simulink model "ObsPertContinuo"  (R2022b)
settings: Solver=ode45  StartTime=0.0  StopTime=700  RelTol=1e-3  EnableMultiTasking=on
settings Model: Creator=adolfobs  LastModifiedBy=adolfo
settings SolverCC: AlgebraicLoopSolver=TrustRegion
settings DataIOCC: LimitDataPoints=on  MaxDataPoints=25000  SaveFormat=Array  SignalLoggingSaveFormat=ModelDataLogs  ReturnWorkspaceOutputs=off
settings OptimizationCC: BlockReduction=off  BooleanDataType=off  InitFltsAndDblsToZero=on  LifeSpan=inf
settings DebuggingCC: SaveWithParameterizedLinksMsg=none  UnderspecifiedInitializationDetection=Classic  MergeDetectMultiDrivingBlocksExec=none  SignalResolutionControl=TryResolveAllWithWarning  MultiTaskDSMMsg=warning  MultiTaskCondExecSysMsg=none  UnconnectedInputMsg=warning  UnconnectedOutputMsg=warning  UnconnectedLineMsg=warning  SFUnexpectedBacktrackingDiag=warning  SFNoUnconditionalDefaultTransitionDiag=warning  SFExecutionAtInitializationDiag=none  SFMachineParentedDataDiag=warning  ArithmeticOperatorsInVariantConditions=warning
settings HardwareCC: ProdBitPerPointer=32  ProdBitPerSizeT=32  ProdBitPerPtrDiffT=32  ProdLargestAtomicFloat=None  ProdIntDivRoundTo=Undefined  ProdEndianess=Unspecified  ProdWordSize=32  ProdHWDeviceType=32-bit Generic  TargetUnknown=on
settings ModelReferenceCC: EnableRefExpFcnMdlSchedulingChecks=on  PropagateSignalLabelsOutOfModel=off
settings SFSimCC: SimUseLocalCustomCode=off  CustomCodeUndefinedFunction=UseInterfaceOnly
settings RTWCC: RTWUseLocalCustomCode=off
settings CodeAppCC: StateflowObjectComments=on
settings GRTTargetCC: TargetFcnLib=ansi_tfl_tmw.mat  TargetLangStandard=C89/C90 (ANSI)  CombineOutputUpdateFcns=off  GRTInterface=on
settings ConfigComp: CovMetricSettings=dw  CovSaveCumulativeToWorkspaceVar=on  CovSaveSingleToWorkspaceVar=on  CovExternalEMLEnable=off

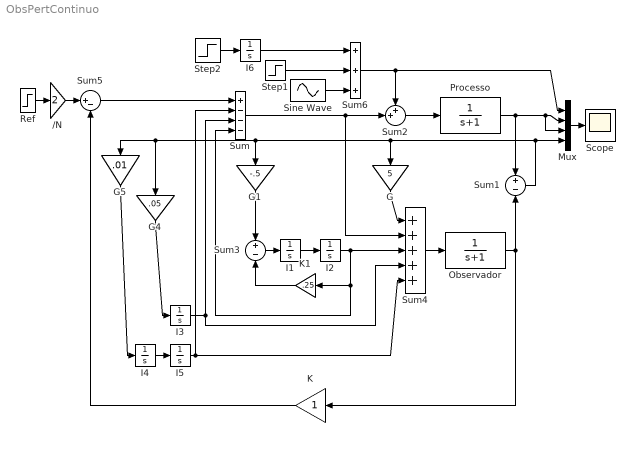
== system ObsPertContinuo ==
  " /N" : Gain  Gain=2  SaturateOnIntegerOverflow=on  OutDataTypeStr=Inherit: Same as input  ParamDataTypeStr=Inherit: Same as input
  G : Gain  Gain=5  SaturateOnIntegerOverflow=on  OutDataTypeStr=Inherit: Same as input  ParamDataTypeStr=Inherit: Same as input
  G1 : Gain  Gain=-.5  SaturateOnIntegerOverflow=on  OutDataTypeStr=Inherit: Same as input  ParamDataTypeStr=Inherit: Same as input
  G4 : Gain  Gain=.05  SaturateOnIntegerOverflow=on  OutDataTypeStr=Inherit: Same as input  ParamDataTypeStr=Inherit: Same as input
  G5 : Gain  Gain=.01  SaturateOnIntegerOverflow=on  OutDataTypeStr=Inherit: Same as input  ParamDataTypeStr=Inherit: Same as input
  I{1..6} (6 alike) : Integrator
  K : Gain  SaturateOnIntegerOverflow=on  OutDataTypeStr=Inherit: Same as input  ParamDataTypeStr=Inherit: Same as input
  K1 : Gain  Gain=.25  SaturateOnIntegerOverflow=on  OutDataTypeStr=Inherit: Same as input  ParamDataTypeStr=Inherit: Same as input
  Mux : Mux
  Observador : TransferFcn  Denominator=[1 1]
  Processo : TransferFcn  Denominator=[1 1]
  Ref : Step  Time=100
  Scope : Scope
  Sine Wave : Sin  Amplitude=.3  Frequency=.5
  Step1 : Step  Time=140  After=.2
  Step2 : Step  Time=400  After=.01
  Sum : Sum  Inputs=+---  InputSameDT=on  SaturateOnIntegerOverflow=on  OutDataTypeStr=Inherit: Same as first input
  Sum1 : Sum  Inputs=+-  InputSameDT=on  SaturateOnIntegerOverflow=on  OutDataTypeStr=Inherit: Same as first input
  Sum2 : Sum  Inputs=++|  InputSameDT=on  SaturateOnIntegerOverflow=on  OutDataTypeStr=Inherit: Same as first input
  Sum3 : Sum  Inputs=+|-  InputSameDT=on  SaturateOnIntegerOverflow=on  OutDataTypeStr=Inherit: Same as first input
  Sum4 : Sum  Inputs=+++++  InputSameDT=on  SaturateOnIntegerOverflow=on  OutDataTypeStr=Inherit: Same as first input
  Sum5 : Sum  Inputs=|+-  InputSameDT=on  SaturateOnIntegerOverflow=on  OutDataTypeStr=Inherit: Same as first input
  Sum6 : Sum  Inputs=+++  InputSameDT=on  SaturateOnIntegerOverflow=on  OutDataTypeStr=Inherit: Same as first input
  wires:
  Sum2/1 -> Processo/1
  Sum/1 -> Sum2/2, Sum4/2
  Mux/1 -> Scope/1
  Sum1/1 -> G/1, G1/1, G4/1, G5/1, Mux/4
  Sum3/1 -> I1/1
  I1/1 -> I2/1
  I2/1 -> Sum4/3, K1/1, Sum/4
  Observador/1 -> Sum1/2, K/1
  Sum4/1 -> Observador/1
  G/1 -> Sum4/1
  G1/1 -> Sum3/1
  Sum5/1 -> Sum/1
  K/1 -> Sum5/2
  Processo/1 -> Sum1/1, Mux/2, Mux/3
  Ref/1 -> " /N"/1
  " /N"/1 -> Sum5/1
  Sum6/1 -> Sum2/1, Mux/1
  I3/1 -> Sum4/4, Sum/3
  G4/1 -> I3/1
  G5/1 -> I4/1
  I4/1 -> I5/1
  I5/1 -> Sum/2, Sum4/5
  Sine Wave/1 -> Sum6/3
  Step1/1 -> Sum6/2
  Step2/1 -> I6/1
  I6/1 -> Sum6/1
  K1/1 -> Sum3/2
